simulink model "uz_codegen"  (R2021a)
settings: Solver=FixedStepDiscrete  StartTime=0.0  StopTime=50  RelTol=1e-3  EnableMultiTasking=on
PreLoadFcn:
  | uz_setCodegenPaths
model workspace (MATLAB code in the model file):
  | cmdLim = Simulink.Parameter;
  | cmdLim.Value = 15;
  | cmdLim.Description = 'Limit for controlling the maximum surface command angle.';
  | cmdLim.Min = 0;
  | cmdLim.Max = 90;
  | cmdLim.DocUnits = 'deg';
  | 
  | dispGain = Simulink.Parameter;
  | dispGain.Value = 0.75;
  | dispGain.Description = 'Gain applied to the displacement error.';
  | dispGain.Min = 0;
  | dispGain.Max = [];
  | dispGain.DocUnits = 'deg/sec/deg';
  | 
  | dispLim = Simulink.Parameter;
  | dispLim.Value = 30;
  | dispLim.Description = 'Limit for controlling the maximum commanded angle.';
  | dispLim.Min = 0;
  | dispLim.Max = 180;
  | dispLim.DocUnits = 'deg';
  | 
  | intGain = Simulink.Parameter;
  | intGain.Value = 0.5;
  | intGain.Description = 'Gain applied to the integral error.';
  | intGain.Min = 0;
  | intGain.Max = [];
  | intGain.DocUnits = 'deg/sec/deg/sec';
  | 
  | intLim = Simulink.Parameter;
  | intLim.Value = 5;
  | intLim.Description = 'Limit for controlling the maximum commanded angle.';
  | intLim.Min = 0;
  | intLim.Max = 90;
  | intLim.DocUnits = 'deg';
  | 
  | rateGain = Simulink.Parameter;
  | rateGain.Value = 2;
  | rateGain.Description = 'Gain applied to the rate error.';
  | rateGain.Min = 0;
  | rateGain.Max = [];
  | rateGain.DocUnits = 'deg/deg/sec';
  | 
  | rateLim = Simulink.Parameter;
  | rateLim.Value = 6;
  | rateLim.Description = 'Limit for controlling the maximum commanded angle.';
  | rateLim.Min = 0;
  | rateLim.Max = 180;
  | rateLim.DocUnits = 'deg/sec';
  | 
  | hdgGain = Simulink.Parameter;
  | hdgGain.Value = 0.015;
values from neighbouring files (symbols this model uses):
  I_max = 100    [PMSM_01_Parameter.m]
  Iq_Intersection_Wb = sqrt(I_max^2 - Id_Intersection_Wb^2)    [Plot_MMPA.m]
  Ki_IdController = R/Ld    (= 3749.81250937)    [PMSM_01_Parameter.m]
  Ki_IqController = R/Lq    (= 2500)    [PMSM_01_Parameter.m]
  Ki_SpeedController = Kp_IqController/(Lq*damping_factor^2)    (= 174.532925199)    [PMSM_01_Parameter.m]
  Ki_TorqueController = 1/(4*T_summe_Torque)    (= 714.285714286)    [PMSM_01_Parameter.m]
  Kp_IdController = Ld*2*pi*BW    (= 0.0670239943087)    [PMSM_01_Parameter.m]
  Kp_IqController = Lq*2*pi*BW    (= 0.100530964915)    [PMSM_01_Parameter.m]
  Kp_SpeedController = Kp_IqController/(Lq*damping_factor*K)    (= 2.90111828368)    [PMSM_01_Parameter.m]
  Kp_TorqueController = T1_Torque/(2*T_summe_Torque)    (= 0.373999125427)    [PMSM_01_Parameter.m]
  Ld = 0.6667*Lq    (= 1.06672e-05)    [PMSM_01_Parameter.m]
  List_Iq_Intersection_Speed = zeros(length(List_wEl_Intersection_Speed),1)    [Plot_MMPA.m]
  List_Iq_Torque = zeros(length(List_M_const),1)    [Plot_MMPA.m]
  List_Iq_Torque_Imax = List_Iq_Torque_Imax(List_Iq_Torque_Imax ~= -1)    [Plot_MMPA.m]
  List_M_const = 0:0.5:10    [Plot_MMPA.m]
  List_M_Imax = List_M_const(List_Iq_Torque_Imax ~= -1)    [Plot_MMPA.m]
  List_wEl_Intersection_Speed = linspace(n_cut,n_max,15)    [Plot_MMPA.m]
  Lq = 16e-6    (= 1.6e-05)    [PMSM_01_Parameter.m]
  n_cut = w_b*30/(pi*zp)    [Plot_MMPA.m]
  psi_pm = 0.0030    (= 0.003)    [PMSM_01_Parameter.m]
  R = 0.040    (= 0.04)    [PMSM_01_Parameter.m]
  T_controller = 1/f_CurrentController    (= 0.0001)    [PMSM_01_Parameter.m]
  T_speedController = T_controller    (= 0.0001)    [PMSM_01_Parameter.m]
  U_DC = 46    [PMSM_01_Parameter.m]
  U_maxDQ = U_DC/sqrt(3)    [PMSM_01_Parameter.m]
  zp = 21    [PMSM_01_Parameter.m]
undefined symbols (not defined in the file or in its folder): denum_Gd_speed, denum_Gd_trq, num_Gd_speed, num_Gd_trq
libraries: pid_lib x8, simulink x7, spsabctodq0Lib x2, spsdq0toAlphaBetaZeroLib x2
(part 1 of 2)
settings Model: RequirementInfo={} %GIDa_fe9045fd_0412_4b6e_8206_617cc20e6fde  FPTRunName=Active  Creator=ts  LastModifiedBy=wilflingti66489
settings SolverCC: AlgebraicLoopSolver=TrustRegion  PositivePriorityOrder=on  AutoInsertRateTranBlk=on
settings DataIOCC: SaveOutput=off  SignalLogging=off  DSMLogging=off  SaveTime=off
settings OptimizationCC: DefaultParameterBehavior=Inlined  UseDivisionForNetSlopeComputation=on  GainParamInheritBuiltInType=on  UseFloatMulNetSlope=on  UseSpecifiedMinMax=on  InlineInvariantSignals=on  PassReuseOutputArgsAs=Individual arguments  NoFixptDivByZeroProtection=on  EfficientFloat2IntCast=on  LifeSpan=1  MaxStackSize=64  OptimizeBlockOrder=speed  DifferentSizesBufferReuse=on  EfficientTunableParamExpr=on
settings DebuggingCC: AllowSymbolicDim=off  SFUnexpectedBacktrackingDiag=warning  SFNoUnconditionalDefaultTransitionDiag=warning  SFExecutionAtInitializationDiag=none  SFMachineParentedDataDiag=warning  ArithmeticOperatorsInVariantConditions=warning
settings HardwareCC: ProdBitPerPointer=32  ProdBitPerSizeT=32  ProdBitPerPtrDiffT=32  ProdLargestAtomicInteger=Long  ProdLargestAtomicFloat=Double  ProdWordSize=32  ProdLongLongMode=on  ProdHWDeviceType=ARM Compatible->ARM Cortex-R  HardwareBoardFeatureSet=SoCBlockset
settings SFSimCC: MATLABDynamicMemAlloc=off
settings RTWCC: SystemTargetFile=ert.tlc  GenCodeOnly=on  TemplateMakefile=ert_default_tmf  GenerateReport=on  BuildConfiguration=Faster Runs  IncludeHyperlinkInReport=on  GenerateCodeMetricsReport=on  CheckMdlBeforeBuild=Warning
settings CodeAppCC: ForceParamTrailComments=on  IgnoreCustomStorageClasses=off  OperatorAnnotations=on  SimulinkDataObjDesc=on  SFDataObjDesc=on  MATLABFcnDesc=on  CustomSymbolStrGlobalVar=rt$N$M  CustomSymbolStrType=$N$M  CustomSymbolStrFcn=$N$M$F  CustomSymbolStrMacro=$N$M  InsertBlockDesc=on  StateflowObjectComments=on  MATLABSourceComments=on  EnableCustomComments=on  ReqsInCode=on
settings ERTTargetCC: TargetLangStandard=C99 (ISO)  CodeReplacementLibrary=GNU C99 extensions  MultiwordLength=2048  IncludeMdlTerminateFcn=off  CombineSignalStateStructs=on  SuppressErrorStatus=on  IncludeFileDelimiter=UseQuote  CodeInterfacePackaging=Reusable function  RemoveResetFunc=off  InlinedParameterPlacement=NonHierarchical  MultiInstanceErrorCode=Warning  RootIOFormat=Part of model data structure  ERTCustomFileTemplate=example_file_process.tlc  GlobalDataDefinition=InSourceFile  GlobalDataReference=InSourceFile  ERTFilePackagingFormat=CompactWithDataFile
settings ConfigComp: CovScope=ReferencedModels  CovSaveName=covdata_rollAP  CovMetricSettings=dcmtrwe  CovHTMLOptions=-sRT=1 -aTS=1 -bRG=1 -bTC=1 -hTR=1 -nFC=0 -scm=1 -bcm=1 -xEv=0  CovSaveCumulativeToWorkspaceVar=on  CovSaveSingleToWorkspaceVar=on  CovCumulativeVarName=covCumulativeData_rollAP  CovReportOnPause=off  CovExternalEMLEnable=off  CovSFcnEnable=off

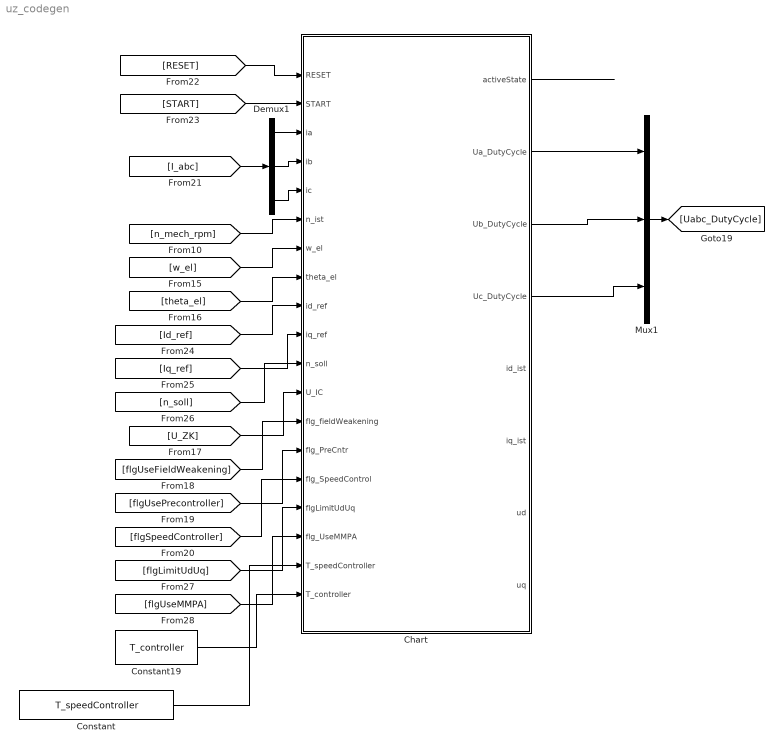
== system uz_codegen ==
  Chart : Stateflow chart  TreatAsAtomicUnit=on
      settings: PortSchema="{\"entries\":[{\"content\":{\"sides\":[{\"content\":{\"connectorIds\":[\"In14\",\"In15\",\"In7\",\"In5\",\"In4\",\"In10\",\"In6\",\"In8\",\"In11\",\"In9\",\"In12\",\"In13\",\"In2\",\"In1\",\"In3\",\"In16\",\"In17\",\"In18\",\"In19\"]},\"type\":\"ConnectorPlacement.EquallySpacedRectSide\",\"uuid\":\"76a4c5fd-8833-454d-a27c-9cb5ddbec7a7\"},{\"content\":{\"connectorIds\":[\"Out2\",\"Out1\",\"Out4\",\"Out3\",\"Out6\",\"Out5\",\"Out8\",\"Out7\"],\"side\":\"RIGHT\"},\"type\":\"ConnectorPlacement.EquallySpacedRectSide\",\"uuid\":\"21c8cff2-6555-410e-8e51-882650c7a948\"},{\"content\":{\"connectorIds\":[],\"side\":\"TOP\"},\"type\":\"ConnectorPlacement.EquallySpacedRectSide\",\"uuid\":\"0c75ee88-c520-42c4-9c42-3a1aac3b64b6\"}]},\"type\":\"ConnectorPlacement.EquallySpacedConnector\",\"uuid\":\"5756a7ca-2edf-4f43-a7f7-e1c56b726d1a\"}],\"packageUris\":[\"http://schema.mathworks.com/mf0/Connector/R2020b\"],\"version\":\"1.0\"}"
  Constant : Constant  Value=T_speedController
  Constant19 : Constant  Value=T_controller
  Demux1 : Demux  Outputs=3
  Mux1 : Mux  Inputs=3
  wires:
  Demux1/3 -> Chart/4(ic)
  [flgUsePrecontroller] -> Chart/1(flg_PreCntr)
  [flgUseMMPA] -> Chart/17(flg_UseMMPA)
  Constant/1 -> Chart/18(T_speedController)
  [flgUseFieldWeakening] -> Chart/2(flg_fieldWeakening)
  Chart/3(Uc_DutyCycle) -> Mux1/3
  [w_el] -> Chart/6(w_el)
  [flgLimitUdUq] -> Chart/16(flgLimitUdUq)
  [n_mech_rpm] -> Chart/10(n_ist)
  [U_ZK] -> Chart/13(U_IC)
  Chart/4(Ub_DutyCycle) -> Mux1/2
  Demux1/1 -> Chart/7(ia)
  Chart/2(activeState) -> ?
  [Iq_ref] -> Chart/9(iq_ref)
  [n_soll] -> Chart/12(n_soll)
  Mux1/1 -> [Uabc_DutyCycle]
  Constant19/1 -> Chart/19(T_controller)
  [theta_el] -> Chart/8(theta_el)
  [flgSpeedController] -> Chart/3(flg_SpeedControl)
  [I_abc] -> Demux1/1
  Chart/1(Ua_DutyCycle) -> Mux1/1
  [START] -> Chart/15(START)
  Demux1/2 -> Chart/5(ib)
  [RESET] -> Chart/14(RESET)
  [Id_ref] -> Chart/11(id_ref)

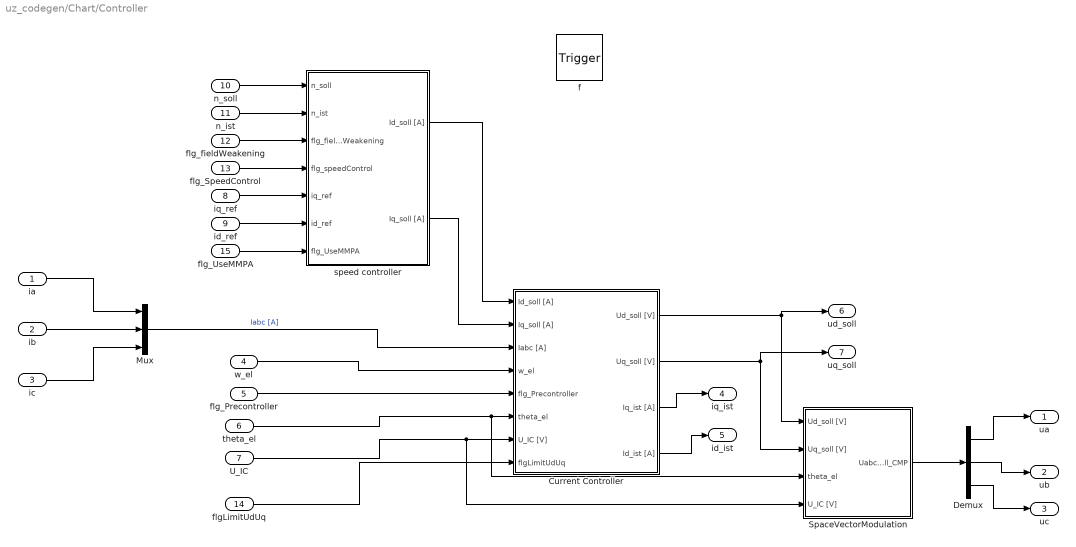
== system uz_codegen/Chart/Controller ==
  ia : Inport  OutDataTypeStr=double  PortDimensions=1
  ib : Inport  Port=2  OutDataTypeStr=double  PortDimensions=1
  ic : Inport  Port=3  OutDataTypeStr=double  PortDimensions=1
  w_el : Inport  Port=4  OutDataTypeStr=double  PortDimensions=1
  flg_Precontroller : Inport  Port=5  OutDataTypeStr=double  PortDimensions=1
  theta_el : Inport  Port=6  OutDataTypeStr=double  PortDimensions=1
  U_IC : Inport  Port=7  OutDataTypeStr=double  PortDimensions=1
  iq_ref : Inport  Port=8  OutDataTypeStr=double  PortDimensions=1
  id_ref : Inport  Port=9  OutDataTypeStr=double  PortDimensions=1
  n_soll : Inport  Port=10  OutDataTypeStr=double  PortDimensions=1
  n_ist : Inport  Port=11  OutDataTypeStr=double  PortDimensions=1
  flg_fieldWeakening : Inport  Port=12  OutDataTypeStr=double  PortDimensions=1
  flg_SpeedControl : Inport  Port=13  OutDataTypeStr=double  PortDimensions=1
  flgLimitUdUq : Inport  Port=14  OutDataTypeStr=double  PortDimensions=1
  flg_UseMMPA : Inport  Port=15  OutDataTypeStr=double  PortDimensions=1
  f : TriggerPort  TriggerType=function-call  VariantControl=(inherit)
      settings: CopyFcn=Stateflow.SLINSF.SimulinkMan.removeBlockPreDeleteFcn  PreDeleteFcn=Stateflow.SLINSF.SimulinkMan.unsafePredeleteFcn
  Current Controller : Subsystem
  Demux : Demux  Outputs=3
  Mux : Mux  Inputs=3
  SpaceVectorModulation : Subsystem
  speed controller : Subsystem
  ua : Outport
  ub : Outport  Port=2
  uc : Outport  Port=3
  iq_ist : Outport  Port=4
  id_ist : Outport  Port=5
  ud_soll : Outport  Port=6
  uq_soll : Outport  Port=7
  wires:
  Current Controller/2(Uq_soll [V]) -> uq_soll/1, SpaceVectorModulation/2(Uq_soll [V])
  speed controller/1(Id_soll [A]) -> Current Controller/1(Id_soll [A])
  Current Controller/1(Ud_soll [V]) -> ud_soll/1, SpaceVectorModulation/1(Ud_soll [V])
  speed controller/2(Iq_soll [A]) -> Current Controller/2(Iq_soll [A])
  SpaceVectorModulation/1(Uabc_soll_CMP) -> Demux/1
  Demux/1 -> ua/1
  Demux/2 -> ub/1
  Demux/3 -> uc/1
  Current Controller/3(Iq_ist [A]) -> iq_ist/1
  Current Controller/4(Id_ist [A]) -> id_ist/1
  ic/1 -> Mux/3
  ib/1 -> Mux/2
  ia/1 -> Mux/1
  Mux/1 -> Current Controller/3(Iabc [A])  "Iabc [A]"
  w_el/1 -> Current Controller/4(w_el)
  flg_Precontroller/1 -> Current Controller/5(flg_Precontroller)
  theta_el/1 -> SpaceVectorModulation/3(theta_el), Current Controller/6(theta_el)
  U_IC/1 -> SpaceVectorModulation/4(U_IC [V]), Current Controller/7(U_IC [V])
  iq_ref/1 -> speed controller/5(iq_ref)
  id_ref/1 -> speed controller/6(id_ref)
  n_soll/1 -> speed controller/1(n_soll)
  n_ist/1 -> speed controller/2(n_ist)
  flg_fieldWeakening/1 -> speed controller/3(flg_fieldWeakening)
  flg_SpeedControl/1 -> speed controller/4(flg_speedControl)
  flgLimitUdUq/1 -> Current Controller/8(flgLimitUdUq)
  flg_UseMMPA/1 -> speed controller/7(flg_UseMMPA)

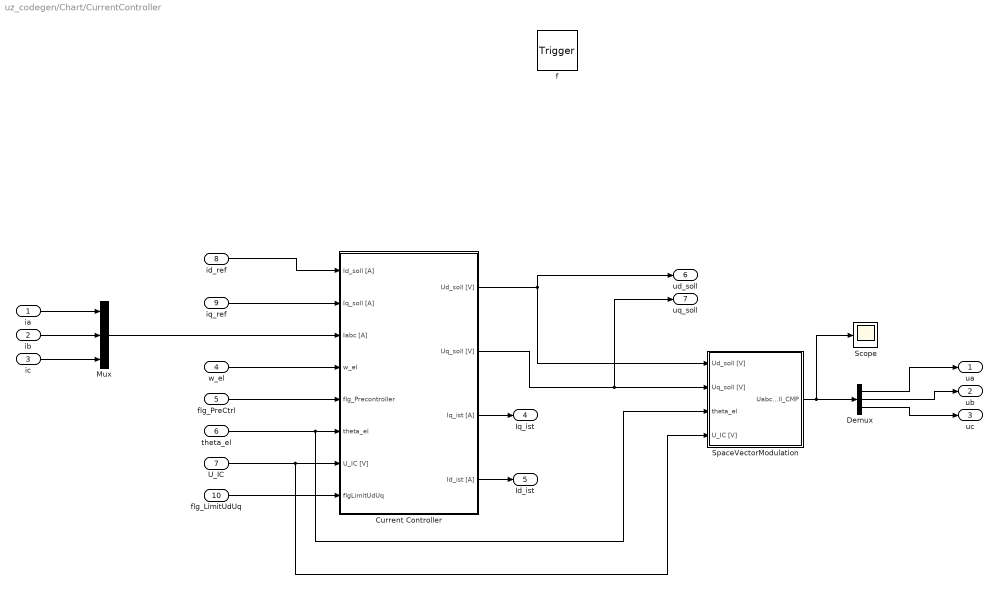
== system uz_codegen/Chart/CurrentController ==
  ia : Inport  OutDataTypeStr=double  PortDimensions=1
  ib : Inport  Port=2  OutDataTypeStr=double  PortDimensions=1
  ic : Inport  Port=3  OutDataTypeStr=double  PortDimensions=1
  w_el : Inport  Port=4  OutDataTypeStr=double  PortDimensions=1
  flg_PreCtrl : Inport  Port=5  OutDataTypeStr=double  PortDimensions=1
  theta_el : Inport  Port=6  OutDataTypeStr=double  PortDimensions=1
  U_IC : Inport  Port=7  OutDataTypeStr=double  PortDimensions=1
  id_ref : Inport  Port=8  OutDataTypeStr=double  PortDimensions=1
  iq_ref : Inport  Port=9  OutDataTypeStr=double  PortDimensions=1
  flg_LimitUdUq : Inport  Port=10  OutDataTypeStr=double  PortDimensions=1
  f : TriggerPort  TriggerType=function-call  VariantControl=(inherit)
      settings: CopyFcn=Stateflow.SLINSF.SimulinkMan.removeBlockPreDeleteFcn  PreDeleteFcn=Stateflow.SLINSF.SimulinkMan.unsafePredeleteFcn
  Current Controller : Subsystem
  Demux : Demux  Outputs=3
  Mux : Mux  Inputs=3
  Scope : Scope
  SpaceVectorModulation : Subsystem
  ua : Outport
  ub : Outport  Port=2
  uc : Outport  Port=3
  Iq_ist : Outport  Port=4
  Id_ist : Outport  Port=5
  ud_soll : Outport  Port=6
  uq_soll : Outport  Port=7
  wires:
  Current Controller/2(Uq_soll [V]) -> uq_soll/1, SpaceVectorModulation/2(Uq_soll [V])
  id_ref/1 -> Current Controller/1(Id_soll [A])
  iq_ref/1 -> Current Controller/2(Iq_soll [A])
  w_el/1 -> Current Controller/4(w_el)
  flg_LimitUdUq/1 -> Current Controller/8(flgLimitUdUq)
  U_IC/1 -> SpaceVectorModulation/4(U_IC [V]), Current Controller/7(U_IC [V])
  theta_el/1 -> SpaceVectorModulation/3(theta_el), Current Controller/6(theta_el)
  flg_PreCtrl/1 -> Current Controller/5(flg_Precontroller)
  ib/1 -> Mux/2
  ia/1 -> Mux/1
  ic/1 -> Mux/3
  Mux/1 -> Current Controller/3(Iabc [A])
  Current Controller/3(Iq_ist [A]) -> Iq_ist/1
  Current Controller/4(Id_ist [A]) -> Id_ist/1
  SpaceVectorModulation/1(Uabc_soll_CMP) -> Scope/1, Demux/1
  Demux/1 -> ua/1
  Demux/2 -> ub/1
  Demux/3 -> uc/1
  Current Controller/1(Ud_soll [V]) -> SpaceVectorModulation/1(Ud_soll [V]), ud_soll/1

== system uz_codegen/Chart/SpeedController ==
  id_ref : Inport  OutDataTypeStr=double  PortDimensions=1
  iq_ref : Inport  Port=2  OutDataTypeStr=double  PortDimensions=1
  n_soll : Inport  Port=3  OutDataTypeStr=double  PortDimensions=1
  n_ist : Inport  Port=4  OutDataTypeStr=double  PortDimensions=1
  flg_fieldWeakening : Inport  Port=5  OutDataTypeStr=double  PortDimensions=1
  flg_UseMMPA : Inport  Port=6  OutDataTypeStr=double  PortDimensions=1
  flg_SpeedControl : Inport  Port=7  OutDataTypeStr=double  PortDimensions=1
  f : TriggerPort  TriggerType=function-call  VariantControl=(inherit)
      settings: CopyFcn=Stateflow.SLINSF.SimulinkMan.removeBlockPreDeleteFcn  PreDeleteFcn=Stateflow.SLINSF.SimulinkMan.unsafePredeleteFcn
  Scope : Scope  NumInputPorts=2
  speed controller : Subsystem
  id_soll : Outport
  iq_soll : Outport  Port=2
  wires:
  flg_SpeedControl/1 -> speed controller/7(flg_speedControl)
  flg_UseMMPA/1 -> speed controller/6(flg_UseMMPA)
  flg_fieldWeakening/1 -> speed controller/5(flg_fieldWeakening)
  n_ist/1 -> speed controller/4(n_ist)
  n_soll/1 -> speed controller/3(n_soll)
  iq_ref/1 -> speed controller/2(iq_ref)
  id_ref/1 -> speed controller/1(id_ref)
  speed controller/1(Id_soll [A]) -> Scope/1, id_soll/1
  speed controller/2(Iq_soll [A]) -> Scope/2, iq_soll/1

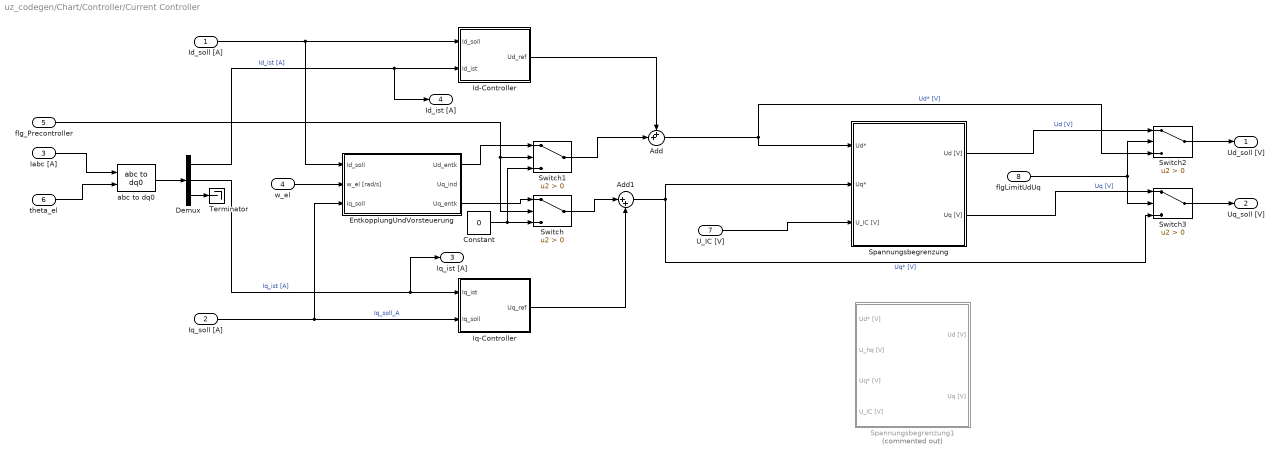
== system uz_codegen/Chart/Controller/Current Controller ==
  Id_soll [A] : Inport
  Iq_soll [A] : Inport  Port=2
  Iabc [A] : Inport  Port=3
  w_el : Inport  Port=4
  flg_Precontroller : Inport  Port=5
  theta_el : Inport  Port=6
  U_IC [V] : Inport  Port=7
  flgLimitUdUq : Inport  Port=8
  Add : Sum  Inputs=++|
  Add1 : Sum  Inputs=|++
  Constant : Constant  Value=0
  Demux : Demux  Outputs=3
  EntkopplungUndVorsteuerung : Subsystem
  Id-Controller : Subsystem
  Iq-Controller : Subsystem
  Spannungsbegrenzung : Subsystem
  Spannungsbegrenzung1 : Subsystem  Commented=on
  Switch{,1..3} (4 alike) : Switch  Criteria=u2 > Threshold
  Terminator : Terminator
  abc to dq0 : spsabctodq0Lib/abc to dq0  Alignment=Aligned with phase A axis
  Ud_soll [V] : Outport
  Uq_soll [V] : Outport  Port=2
  Iq_ist [A] : Outport  Port=3
  Id_ist [A] : Outport  Port=4
  wires:
  Add1/1 -> Switch3/3, Spannungsbegrenzung/2(Uq*)  "Uq* [V]"
  Add/1 -> Switch2/3, Spannungsbegrenzung/1(Ud*)  "Ud* [V]"
  Id_soll [A]/1 -> EntkopplungUndVorsteuerung/1(Id_soll), Id-Controller/1(Id_soll)
  Iabc [A]/1 -> abc to dq0/1
  theta_el/1 -> abc to dq0/2
  abc to dq0/1 -> Demux/1
  Demux/1 -> Id_ist [A]/1, Id-Controller/2(Id_ist)  "Id_ist [A]"
  Demux/2 -> Iq_ist [A]/1, Iq-Controller/1(Iq_ist)  "Iq_ist [A]"
  Demux/3 -> Terminator/1
  w_el/1 -> EntkopplungUndVorsteuerung/2(w_el [rad/s])
  EntkopplungUndVorsteuerung/3(Uq_entk) -> Switch/1
  EntkopplungUndVorsteuerung/1(Ud_entk) -> Switch1/1
  Constant/1 -> Switch1/3, Switch/3
  flg_Precontroller/1 -> Switch/2, Switch1/2
  Iq-Controller/1(Uq_ref) -> Add1/2
  Iq_soll [A]/1 -> EntkopplungUndVorsteuerung/3(Iq_soll), Iq-Controller/2(Iq_soll)  "Iq_soll_A"
  U_IC [V]/1 -> Spannungsbegrenzung/3(U_IC [V])
  Spannungsbegrenzung/1(Ud [V]) -> Switch2/1  "Ud [V]"
  Spannungsbegrenzung/2(Uq [V]) -> Switch3/1  "Uq [V]"
  Switch1/1 -> Add/2
  Switch/1 -> Add1/1
  Id-Controller/1(Ud_ref) -> Add/1
  Switch2/1 -> Ud_soll [V]/1
  Switch3/1 -> Uq_soll [V]/1
  flgLimitUdUq/1 -> Switch3/2, Switch2/2

== system uz_codegen/Chart/Controller/SpaceVectorModulation ==
  Ud_soll [V] : Inport
  Uq_soll [V] : Inport  Port=2
  theta_el : Inport  Port=3
  U_IC [V] : Inport  Port=4
  Constant : Constant  Value=0
  Demux : Demux  Outputs=3
  Mux : Mux  Inputs=3
  Mux2 : Mux  Inputs=3
  SpaceVectorModulation : MATLAB Function  TreatAsAtomicUnit=on
  Terminator : Terminator
  dq0 to Alpha-Beta-Zero : spsdq0toAlphaBetaZeroLib/dq0 to Alpha-Beta-Zero  Alignment=Aligned with phase A axis
      settings: SourceProductBaseCode=PS
  Uabc_soll_CMP : Outport
  wires:
  Ud_soll [V]/1 -> Mux/1
  Uq_soll [V]/1 -> Mux/2
  Constant/1 -> Mux/3
  Mux/1 -> dq0 to Alpha-Beta-Zero/1  "Udq0 [V]"
  theta_el/1 -> dq0 to Alpha-Beta-Zero/2
  Demux/1 -> SpaceVectorModulation/1(u_alpha)
  Demux/2 -> SpaceVectorModulation/2(u_beta)
  Demux/3 -> Terminator/1
  SpaceVectorModulation/1(u_a) -> Mux2/1
  SpaceVectorModulation/2(u_b) -> Mux2/2
  SpaceVectorModulation/3(u_c) -> Mux2/3
  dq0 to Alpha-Beta-Zero/1 -> Demux/1  "UalphaBeta [V]"
  Mux2/1 -> Uabc_soll_CMP/1  "Uabc_soll_CMP"
  U_IC [V]/1 -> SpaceVectorModulation/3(U_ZK)

== system uz_codegen/Chart/Controller/speed controller ==
  n_soll : Inport
  n_ist : Inport  Port=2
  flg_fieldWeakening : Inport  Port=3
  flg_speedControl : Inport  Port=4
  iq_ref : Inport  Port=5
  id_ref : Inport  Port=6
  flg_UseMMPA : Inport  Port=7
  MMPA_Controller : Subsystem
  Subsystem : Subsystem
  Switch : Switch  Criteria=u2 > Threshold
  Switch1 : Switch  Criteria=u2 > Threshold
  Id_soll [A] : Outport
  Iq_soll [A] : Outport  Port=2
  wires:
  flg_fieldWeakening/1 -> Subsystem/1(flg_fieldWeakening)
  id_ref/1 -> MMPA_Controller/4(id_ref), Subsystem/2(id_ref)
  flg_speedControl/1 -> MMPA_Controller/1(flg_speedControl), Subsystem/4(flg_speedControl)
  n_ist/1 -> MMPA_Controller/3(n_ist), Subsystem/5(n_ist)
  iq_ref/1 -> MMPA_Controller/5(iq_ref), Subsystem/6(iq_ref)
  Subsystem/1(id_soll) -> Switch/3
  Subsystem/2(iq_soll) -> Switch1/3
  MMPA_Controller/1(id_soll) -> Switch/1
  Switch/1 -> Id_soll [A]/1
  Switch1/1 -> Iq_soll [A]/1
  MMPA_Controller/2(Iq_soll) -> Switch1/1
  flg_UseMMPA/1 -> Switch/2, Switch1/2
  n_soll/1 -> MMPA_Controller/2(n_soll), Subsystem/3(n_soll)

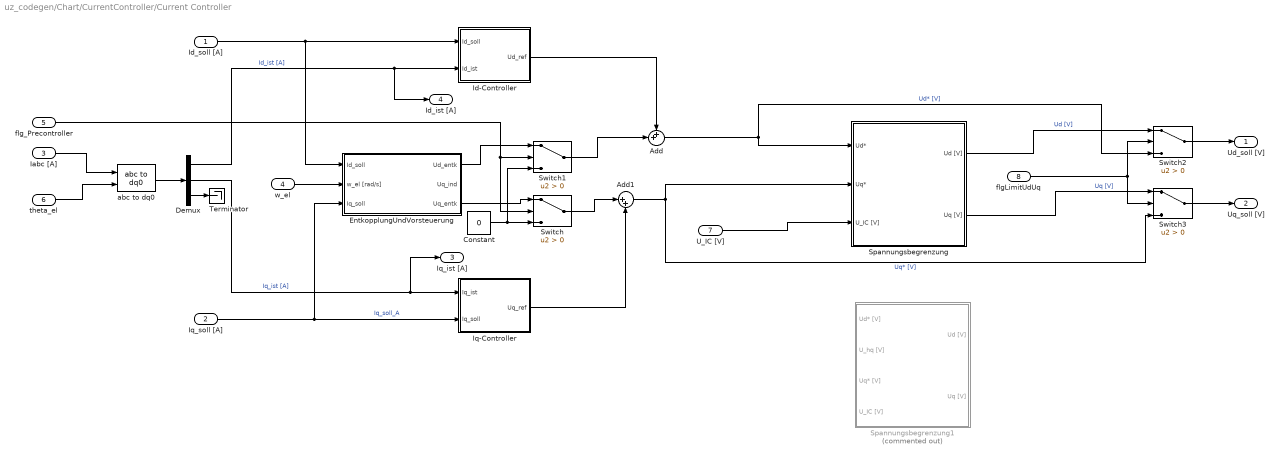
== system uz_codegen/Chart/CurrentController/Current Controller ==
  Id_soll [A] : Inport
  Iq_soll [A] : Inport  Port=2
  Iabc [A] : Inport  Port=3
  w_el : Inport  Port=4
  flg_Precontroller : Inport  Port=5
  theta_el : Inport  Port=6
  U_IC [V] : Inport  Port=7
  flgLimitUdUq : Inport  Port=8
  Add : Sum  Inputs=++|
  Add1 : Sum  Inputs=|++
  Constant : Constant  Value=0
  Demux : Demux  Outputs=3
  EntkopplungUndVorsteuerung : Subsystem
  Id-Controller : Subsystem
  Iq-Controller : Subsystem
  Spannungsbegrenzung : Subsystem
  Spannungsbegrenzung1 : Subsystem  Commented=on
  Switch{,1..3} (4 alike) : Switch  Criteria=u2 > Threshold
  Terminator : Terminator
  abc to dq0 : spsabctodq0Lib/abc to dq0  Alignment=Aligned with phase A axis
  Ud_soll [V] : Outport
  Uq_soll [V] : Outport  Port=2
  Iq_ist [A] : Outport  Port=3
  Id_ist [A] : Outport  Port=4
  wires:
  Add1/1 -> Switch3/3, Spannungsbegrenzung/2(Uq*)  "Uq* [V]"
  Add/1 -> Switch2/3, Spannungsbegrenzung/1(Ud*)  "Ud* [V]"
  Id_soll [A]/1 -> EntkopplungUndVorsteuerung/1(Id_soll), Id-Controller/1(Id_soll)
  Iabc [A]/1 -> abc to dq0/1
  theta_el/1 -> abc to dq0/2
  abc to dq0/1 -> Demux/1
  Demux/1 -> Id_ist [A]/1, Id-Controller/2(Id_ist)  "Id_ist [A]"
  Demux/2 -> Iq_ist [A]/1, Iq-Controller/1(Iq_ist)  "Iq_ist [A]"
  Demux/3 -> Terminator/1
  w_el/1 -> EntkopplungUndVorsteuerung/2(w_el [rad/s])
  EntkopplungUndVorsteuerung/3(Uq_entk) -> Switch/1
  EntkopplungUndVorsteuerung/1(Ud_entk) -> Switch1/1
  Constant/1 -> Switch1/3, Switch/3
  flg_Precontroller/1 -> Switch/2, Switch1/2
  Iq-Controller/1(Uq_ref) -> Add1/2
  Iq_soll [A]/1 -> EntkopplungUndVorsteuerung/3(Iq_soll), Iq-Controller/2(Iq_soll)  "Iq_soll_A"
  U_IC [V]/1 -> Spannungsbegrenzung/3(U_IC [V])
  Spannungsbegrenzung/1(Ud [V]) -> Switch2/1  "Ud [V]"
  Spannungsbegrenzung/2(Uq [V]) -> Switch3/1  "Uq [V]"
  Switch1/1 -> Add/2
  Switch/1 -> Add1/1
  Id-Controller/1(Ud_ref) -> Add/1
  Switch2/1 -> Ud_soll [V]/1
  Switch3/1 -> Uq_soll [V]/1
  flgLimitUdUq/1 -> Switch3/2, Switch2/2

== system uz_codegen/Chart/CurrentController/SpaceVectorModulation ==
  Ud_soll [V] : Inport
  Uq_soll [V] : Inport  Port=2
  theta_el : Inport  Port=3
  U_IC [V] : Inport  Port=4
  Constant : Constant  Value=0
  Demux : Demux  Outputs=3
  Mux : Mux  Inputs=3
  Mux2 : Mux  Inputs=3
  SpaceVectorModulation : MATLAB Function  TreatAsAtomicUnit=on
  Terminator : Terminator
  dq0 to Alpha-Beta-Zero : spsdq0toAlphaBetaZeroLib/dq0 to Alpha-Beta-Zero  Alignment=Aligned with phase A axis
      settings: SourceProductBaseCode=PS
  Uabc_soll_CMP : Outport
  wires:
  Ud_soll [V]/1 -> Mux/1
  Uq_soll [V]/1 -> Mux/2
  Constant/1 -> Mux/3
  Mux/1 -> dq0 to Alpha-Beta-Zero/1  "Udq0 [V]"
  theta_el/1 -> dq0 to Alpha-Beta-Zero/2
  Demux/1 -> SpaceVectorModulation/1(u_alpha)
  Demux/2 -> SpaceVectorModulation/2(u_beta)
  Demux/3 -> Terminator/1
  SpaceVectorModulation/1(u_a) -> Mux2/1
  SpaceVectorModulation/2(u_b) -> Mux2/2
  SpaceVectorModulation/3(u_c) -> Mux2/3
  dq0 to Alpha-Beta-Zero/1 -> Demux/1  "UalphaBeta [V]"
  Mux2/1 -> Uabc_soll_CMP/1  "Uabc_soll_CMP"
  U_IC [V]/1 -> SpaceVectorModulation/3(U_ZK)

== system uz_codegen/Chart/SpeedController/speed controller ==
  id_ref : Inport
  iq_ref : Inport  Port=2
  n_soll : Inport  Port=3
  n_ist : Inport  Port=4
  flg_fieldWeakening : Inport  Port=5
  flg_UseMMPA : Inport  Port=6
  flg_speedControl : Inport  Port=7
  MMPA_Controller : Subsystem
  Subsystem : Subsystem
  Switch : Switch  Criteria=u2 > Threshold
  Switch1 : Switch  Criteria=u2 > Threshold
  Id_soll [A] : Outport
  Iq_soll [A] : Outport  Port=2
  wires:
  flg_fieldWeakening/1 -> Subsystem/1(flg_fieldWeakening)
  id_ref/1 -> MMPA_Controller/4(id_ref), Subsystem/2(id_ref)
  flg_speedControl/1 -> MMPA_Controller/1(flg_speedControl), Subsystem/4(flg_speedControl)
  n_ist/1 -> MMPA_Controller/3(n_ist), Subsystem/5(n_ist)
  iq_ref/1 -> MMPA_Controller/5(iq_ref), Subsystem/6(iq_ref)
  Subsystem/1(id_soll) -> Switch/3
  Subsystem/2(iq_soll) -> Switch1/3
  MMPA_Controller/1(id_soll) -> Switch/1
  Switch/1 -> Id_soll [A]/1
  Switch1/1 -> Iq_soll [A]/1
  MMPA_Controller/2(Iq_soll) -> Switch1/1
  flg_UseMMPA/1 -> Switch/2, Switch1/2
  n_soll/1 -> MMPA_Controller/2(n_soll), Subsystem/3(n_soll)

== system uz_codegen/Chart/Controller/Current Controller/EntkopplungUndVorsteuerung ==
  Id_soll : Inport
  w_el [rad/s] : Inport  Port=2
  Iq_soll : Inport  Port=3
  Add : Sum
  Constant : Constant  Value=psi_pm
  Gain1 : Gain  Gain=-Lq
  Gain2 : Gain  Gain=Ld
  Product : Product
  Product1 : Product
  Product2 : Product
  Ud_entk : Outport
  Uq_ind : Outport  Port=2
  Uq_entk : Outport  Port=3
  wires:
  w_el [rad/s]/1 -> Product2/2, Product1/2, Product/1  "w_el [rad/s]"
  Iq_soll/1 -> Gain1/1
  Gain1/1 -> Product/2
  Product/1 -> Ud_entk/1  "-w_el * Iq * Lq"
  Id_soll/1 -> Gain2/1
  Gain2/1 -> Add/2
  Constant/1 -> Product2/1, Add/1
  Add/1 -> Product1/1
  Product1/1 -> Uq_entk/1  "w_el * (psi_pm + Ld * Id)"
  Product2/1 -> Uq_ind/1

== system uz_codegen/Chart/Controller/Current Controller/Id-Controller ==
  Id_soll : Inport
  Id_ist : Inport  Port=2
  PID Controller : pid_lib/PID Controller  Controller=PI  Form=Ideal  TimeDomain=Discrete-time  UseExternalTs=off  SampleTime=-1  IntegratorMethod=Forward Euler  FilterMethod=Forward Euler  ControllerParametersSource=internal  P=Kp_IdController  I=Ki_IdController  D=0  UseFilter=on  N=100  TunerSelectOption=Transfer Function Based (PID Tuner App)  InitialConditionSource=internal  InitialConditionForIntegrator=0  InitialConditionForFilter=0  DifferentiatorICPrevScaledInput=0  ExternalReset=none  TrackingMode=off  Kt=1  LimitOutput=on  SatLimitsSource=internal  UpperSaturationLimit=U_maxDQ  LowerSaturationLimit=-U_maxDQ  LinearizeAsGain=on  AntiWindupMode=clamping  Kb=1  POutMin=[]  POutMax=[]  IOutMin=[]  IOutMax=[]  DOutMin=[]  DOutMax=[]  NOutMin=[]  NOutMax=[]  SumOutMin=[]  SumOutMax=[]  SaturationOutMin=[]  SaturationOutMax=[]  PParamMin=[]  PParamMax=[]  IParamMin=[]  IParamMax=[]  DParamMin=[]  DParamMax=[]  NParamMin=[]  NParamMax=[]  KbParamMin=[]  KbParamMax=[]  KtParamMin=[]  KtParamMax=[]  KbOutMin=[]  KbOutMax=[]  KtOutMin=[]  KtOutMax=[]  IntegratorOutMin=[]  IntegratorOutMax=[]  FilterOutMin=[]  FilterOutMax=[]  SumI1OutMin=[]  SumI1OutMax=[]  SumI2OutMin=[]  SumI2OutMax=[]  SumI3OutMin=[]  SumI3OutMax=[]  SumI4OutMin=[]  SumI4OutMax=[]  SumDOutMin=[]  SumDOutMax=[]  DifferentiatorOutMin=[]  DifferentiatorOutMax=[]  FilterDiffOutCoefMin=[]  FilterDiffOutCoefMax=[]  ReciprocalOutMin=[]  ReciprocalOutMax=[]  SumDenOutMin=[]  SumDenOutMax=[]  SumNumOutMin=[]  SumNumOutMax=[]  DivideOutMin=[]  DivideOutMax=[]  UdiffTsProdOutMin=[]  UdiffTsProdOutMax=[]  NTsProdOutMin=[]  NTsProdOutMax=[]  UintegralTsProdOutMin=[]  UintegralTsProdOutMax=[]  UngainTsProdOutMin=[]  UngainTsProdOutMax=[]  IntegratorContinuousStateAttributes=''  IntegratorStateMustResolveToSignalObject=off  IntegratorRTWStateStorageClass=Auto  FilterContinuousStateAttributes=''  FilterStateMustResolveToSignalObject=off  FilterRTWStateStorageClass=Auto  ParallelPVariant=Passthrough  IdealPVariant=InternalParameters  IVariant=InternalParameters  DVariant=Disabled  IntegratorVariant=Discrete  SatVariant=Enabled  AWVariant=DiscClampingIdeal  PCopyVariant=InternalParamsIdeal  TRVariant=Disabled  FdbkBlocksVariant=Forward  IdealPFdbkVariant=Disabled  SatFdbkVariant=Disabled  DerivativeFilterVariant=Disabled  NVariant=Disabled  NCopyVariant=Disabled_SignalSpec  FilterICVariant=Disabled  IntegratorICVariant=InternalICs  ExternalResetVariant=Disabled  TRSumVariant=Passthrough  SumFdbkVariant=Disabled  SumVariant=Sum_PI  TsampFilterVariant=InternalTs  TsampNgainVariant=Passthrough  TsampIntegralVariant=Passthrough  ExternalSaturationOutDataTypeStr=Inherit: Same as second input
  Scope : Scope  NumInputPorts=2
  Subtract : Sum  Inputs=|+-
  Ud_ref : Outport
  wires:
  Subtract/1 -> PID Controller/1  "error"
  Id_soll/1 -> Scope/1, Subtract/1  "id_soll"
  Id_ist/1 -> Scope/2, Subtract/2  "id_ist"
  PID Controller/1 -> Ud_ref/1

== system uz_codegen/Chart/Controller/Current Controller/Iq-Controller ==
  Iq_ist : Inport
  Iq_soll : Inport  Port=2
  PID Controller : pid_lib/PID Controller  Controller=PI  Form=Ideal  TimeDomain=Discrete-time  UseExternalTs=off  SampleTime=-1  IntegratorMethod=Forward Euler  FilterMethod=Forward Euler  ControllerParametersSource=internal  P=Kp_IqController  I=Ki_IqController  D=0  UseFilter=on  N=100  TunerSelectOption=Transfer Function Based (PID Tuner App)  InitialConditionSource=internal  InitialConditionForIntegrator=0  InitialConditionForFilter=0  DifferentiatorICPrevScaledInput=0  ExternalReset=none  TrackingMode=off  Kt=1  LimitOutput=on  SatLimitsSource=internal  UpperSaturationLimit=U_maxDQ  LowerSaturationLimit=-U_maxDQ  LinearizeAsGain=on  AntiWindupMode=clamping  Kb=1  POutMin=[]  POutMax=[]  IOutMin=[]  IOutMax=[]  DOutMin=[]  DOutMax=[]  NOutMin=[]  NOutMax=[]  SumOutMin=[]  SumOutMax=[]  SaturationOutMin=[]  SaturationOutMax=[]  PParamMin=[]  PParamMax=[]  IParamMin=[]  IParamMax=[]  DParamMin=[]  DParamMax=[]  NParamMin=[]  NParamMax=[]  KbParamMin=[]  KbParamMax=[]  KtParamMin=[]  KtParamMax=[]  KbOutMin=[]  KbOutMax=[]  KtOutMin=[]  KtOutMax=[]  IntegratorOutMin=[]  IntegratorOutMax=[]  FilterOutMin=[]  FilterOutMax=[]  SumI1OutMin=[]  SumI1OutMax=[]  SumI2OutMin=[]  SumI2OutMax=[]  SumI3OutMin=[]  SumI3OutMax=[]  SumI4OutMin=[]  SumI4OutMax=[]  SumDOutMin=[]  SumDOutMax=[]  DifferentiatorOutMin=[]  DifferentiatorOutMax=[]  FilterDiffOutCoefMin=[]  FilterDiffOutCoefMax=[]  ReciprocalOutMin=[]  ReciprocalOutMax=[]  SumDenOutMin=[]  SumDenOutMax=[]  SumNumOutMin=[]  SumNumOutMax=[]  DivideOutMin=[]  DivideOutMax=[]  UdiffTsProdOutMin=[]  UdiffTsProdOutMax=[]  NTsProdOutMin=[]  NTsProdOutMax=[]  UintegralTsProdOutMin=[]  UintegralTsProdOutMax=[]  UngainTsProdOutMin=[]  UngainTsProdOutMax=[]  IntegratorContinuousStateAttributes=''  IntegratorStateMustResolveToSignalObject=off  IntegratorRTWStateStorageClass=Auto  FilterContinuousStateAttributes=''  FilterStateMustResolveToSignalObject=off  FilterRTWStateStorageClass=Auto  ParallelPVariant=Passthrough  IdealPVariant=InternalParameters  IVariant=InternalParameters  DVariant=Disabled  IntegratorVariant=Discrete  SatVariant=Enabled  AWVariant=DiscClampingIdeal  PCopyVariant=InternalParamsIdeal  TRVariant=Disabled  FdbkBlocksVariant=Forward  IdealPFdbkVariant=Disabled  SatFdbkVariant=Disabled  DerivativeFilterVariant=Disabled  NVariant=Disabled  NCopyVariant=Disabled_SignalSpec  FilterICVariant=Disabled  IntegratorICVariant=InternalICs  ExternalResetVariant=Disabled  TRSumVariant=Passthrough  SumFdbkVariant=Disabled  SumVariant=Sum_PI  TsampFilterVariant=InternalTs  TsampNgainVariant=Passthrough  TsampIntegralVariant=Passthrough  ExternalSaturationOutDataTypeStr=Inherit: Same as second input
  Scope : Scope  NumInputPorts=2
  Subtract : Sum  Inputs=|+-
  Uq_ref : Outport
  wires:
  Subtract/1 -> PID Controller/1  "error"
  Iq_soll/1 -> Scope/1, Subtract/1  "iq_soll"
  Iq_ist/1 -> Scope/2, Subtract/2  "iq_ist"
  PID Controller/1 -> Uq_ref/1

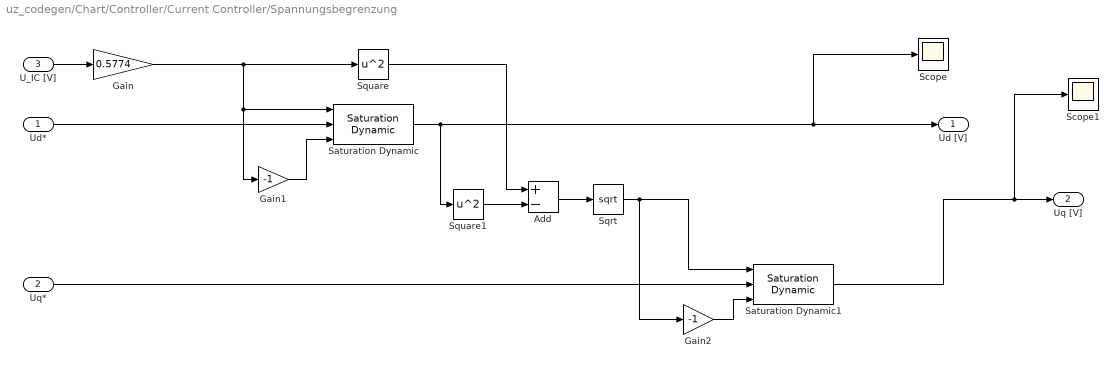
== system uz_codegen/Chart/Controller/Current Controller/Spannungsbegrenzung ==
  Ud* : Inport
  Uq* : Inport  Port=2
  U_IC [V] : Inport  Port=3
  Add : Sum  Inputs=+-
  Gain : Gain  Gain=0.5774
  Gain1 : Gain  Gain=-1
  Gain2 : Gain  Gain=-1
  Saturation Dynamic : simulink/Discontinuities/Saturation Dynamic  OutMin=[]  OutMax=[]  OutDataTypeStr=Inherit: Same as second input  OutDataType=fixdt(1, 16)  OutScaling=2^-10  DoSatur=off
  Saturation Dynamic1 : simulink/Discontinuities/Saturation Dynamic  OutMin=[]  OutMax=[]  OutDataTypeStr=Inherit: Same as second input  OutDataType=fixdt(1, 16)  OutScaling=2^-10  DoSatur=off
  Scope : Scope
  Scope1 : Scope
  Sqrt : Sqrt  SaturateOnIntegerOverflow=on
  Square : Math  Operator=square  SaturateOnIntegerOverflow=on
  Square1 : Math  Operator=square  SaturateOnIntegerOverflow=on
  Ud [V] : Outport
  Uq [V] : Outport  Port=2
  wires:
  Gain2/1 -> Saturation Dynamic1/3
  Add/1 -> Sqrt/1
  Square/1 -> Add/1
  Sqrt/1 -> Gain2/1, Saturation Dynamic1/1
  Saturation Dynamic/1 -> Scope/1, Ud [V]/1, Square1/1
  Saturation Dynamic1/1 -> Scope1/1, Uq [V]/1
  Gain1/1 -> Saturation Dynamic/3
  Uq*/1 -> Saturation Dynamic1/2
  U_IC [V]/1 -> Gain/1
  Gain/1 -> Square/1, Saturation Dynamic/1, Gain1/1
  Square1/1 -> Add/2
  Ud*/1 -> Saturation Dynamic/2

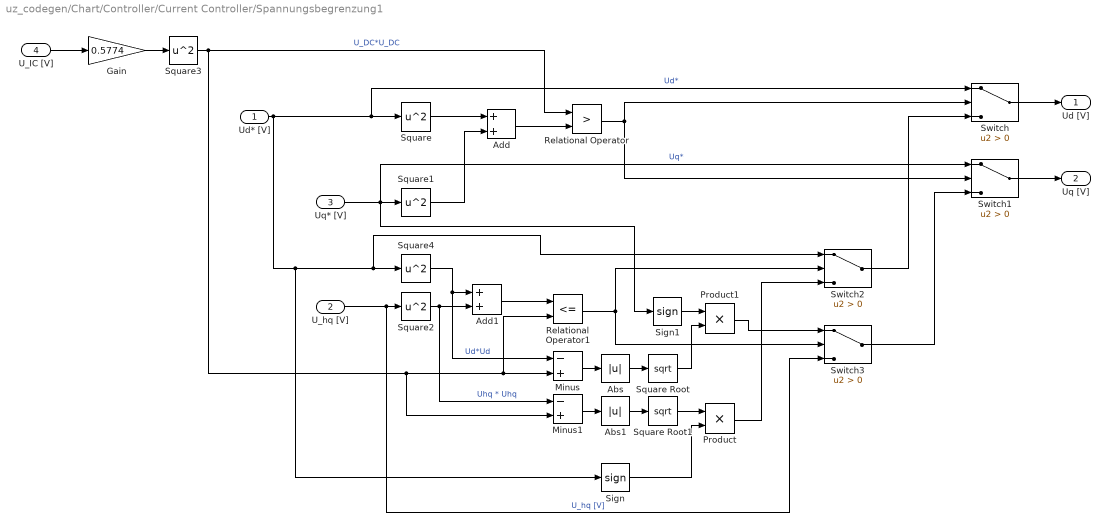
== system uz_codegen/Chart/Controller/Current Controller/Spannungsbegrenzung1 ==
  Ud* [V] : Inport
  U_hq [V] : Inport  Port=2
  Uq* [V] : Inport  Port=3
  U_IC [V] : Inport  Port=4
  Abs : Abs
  Abs1 : Abs
  Add : Sum
  Add1 : Sum
  Gain : Gain  Gain=0.5774
  Minus : Sum  Inputs=-+
  Minus1 : Sum  Inputs=-+
  Product : Product
  Product1 : Product
  Relational Operator : RelationalOperator  Operator=>  OutDataTypeStr=boolean  RndMeth=Simplest
  Relational Operator1 : RelationalOperator  Operator=<=  OutDataTypeStr=boolean  RndMeth=Simplest
  Sign : Signum
  Sign1 : Signum
  Square{,1..4} (5 alike) : Math  Operator=square  SaturateOnIntegerOverflow=on
  Square Root : Sqrt  SaturateOnIntegerOverflow=on
  Square Root1 : Sqrt  SaturateOnIntegerOverflow=on
  Switch{,1..3} (4 alike) : Switch  Criteria=u2 > Threshold
  Ud [V] : Outport
  Uq [V] : Outport  Port=2
  wires:
  Ud* [V]/1 -> Sign/1, Switch2/1, Square4/1, Switch/1, Square/1  "Ud*"
  Uq* [V]/1 -> Switch1/1, Sign1/1, Square1/1  "Uq*"
  U_hq [V]/1 -> Switch3/3, Square2/1  "U_hq [V]"
  U_IC [V]/1 -> Gain/1
  Square1/1 -> Add/2
  Square/1 -> Add/1
  Square3/1 -> Minus1/2, Minus/2, Relational Operator1/2, Relational Operator/1  "U_DC*U_DC"
  Add/1 -> Relational Operator/2
  Switch/1 -> Ud [V]/1
  Relational Operator/1 -> Switch1/2, Switch/2
  Switch1/1 -> Uq [V]/1
  Square2/1 -> Minus1/1, Add1/2  "Uhq * Uhq"
  Square4/1 -> Minus/1, Add1/1  "Ud*Ud"
  Add1/1 -> Relational Operator1/1
  Relational Operator1/1 -> Switch2/2, Switch3/2
  Switch2/1 -> Switch/3
  Switch3/1 -> Switch1/3
  Minus/1 -> Abs/1
  Square Root/1 -> Product1/2
  Minus1/1 -> Abs1/1
  Square Root1/1 -> Product/1
  Abs1/1 -> Square Root1/1
  Abs/1 -> Square Root/1
  Gain/1 -> Square3/1
  Sign/1 -> Product/2
  Product/1 -> Switch2/3
  Sign1/1 -> Product1/1
  Product1/1 -> Switch3/1

== system uz_codegen/Chart/Controller/speed controller/MMPA_Controller ==
  flg_speedControl : Inport
  n_soll : Inport  Port=2
  n_ist : Inport  Port=3
  id_ref : Inport  Port=4
  iq_ref : Inport  Port=5
  Discrete Transfer Fcn : DiscreteTransferFcn  Numerator=num_Gd_trq  Denominator=denum_Gd_trq
  PID Controller : pid_lib/PID Controller  Controller=PI  Form=Ideal  TimeDomain=Discrete-time  UseExternalTs=off  SampleTime=-1  IntegratorMethod=Forward Euler  FilterMethod=Forward Euler  ControllerParametersSource=internal  P=Kp_TorqueController  I=Ki_TorqueController  D=0  UseFilter=on  N=100  TunerSelectOption=Transfer Function Based (PID Tuner App)  InitialConditionSource=internal  InitialConditionForIntegrator=0  InitialConditionForFilter=0  DifferentiatorICPrevScaledInput=0  ExternalReset=none  TrackingMode=off  Kt=1  LimitOutput=on  SatLimitsSource=internal  UpperSaturationLimit=8  LowerSaturationLimit=-8  LinearizeAsGain=on  AntiWindupMode=clamping  Kb=1  POutMin=[]  POutMax=[]  IOutMin=[]  IOutMax=[]  DOutMin=[]  DOutMax=[]  NOutMin=[]  NOutMax=[]  SumOutMin=[]  SumOutMax=[]  SaturationOutMin=[]  SaturationOutMax=[]  PParamMin=[]  PParamMax=[]  IParamMin=[]  IParamMax=[]  DParamMin=[]  DParamMax=[]  NParamMin=[]  NParamMax=[]  KbParamMin=[]  KbParamMax=[]  KtParamMin=[]  KtParamMax=[]  KbOutMin=[]  KbOutMax=[]  KtOutMin=[]  KtOutMax=[]  IntegratorOutMin=[]  IntegratorOutMax=[]  FilterOutMin=[]  FilterOutMax=[]  SumI1OutMin=[]  SumI1OutMax=[]  SumI2OutMin=[]  SumI2OutMax=[]  SumI3OutMin=[]  SumI3OutMax=[]  SumI4OutMin=[]  SumI4OutMax=[]  SumDOutMin=[]  SumDOutMax=[]  DifferentiatorOutMin=[]  DifferentiatorOutMax=[]  FilterDiffOutCoefMin=[]  FilterDiffOutCoefMax=[]  ReciprocalOutMin=[]  ReciprocalOutMax=[]  SumDenOutMin=[]  SumDenOutMax=[]  SumNumOutMin=[]  SumNumOutMax=[]  DivideOutMin=[]  DivideOutMax=[]  UdiffTsProdOutMin=[]  UdiffTsProdOutMax=[]  NTsProdOutMin=[]  NTsProdOutMax=[]  UintegralTsProdOutMin=[]  UintegralTsProdOutMax=[]  UngainTsProdOutMin=[]  UngainTsProdOutMax=[]  IntegratorContinuousStateAttributes=''  IntegratorStateMustResolveToSignalObject=off  IntegratorRTWStateStorageClass=Auto  FilterContinuousStateAttributes=''  FilterStateMustResolveToSignalObject=off  FilterRTWStateStorageClass=Auto  ParallelPVariant=Passthrough  IdealPVariant=InternalParameters  IVariant=InternalParameters  DVariant=Disabled  IntegratorVariant=Discrete  SatVariant=Enabled  AWVariant=DiscClampingIdeal  PCopyVariant=InternalParamsIdeal  TRVariant=Disabled  FdbkBlocksVariant=Forward  IdealPFdbkVariant=Disabled  SatFdbkVariant=Disabled  DerivativeFilterVariant=Disabled  NVariant=Disabled  NCopyVariant=Disabled_SignalSpec  FilterICVariant=Disabled  IntegratorICVariant=InternalICs  ExternalResetVariant=Disabled  TRSumVariant=Passthrough  SumFdbkVariant=Disabled  SumVariant=Sum_PI  TsampFilterVariant=InternalTs  TsampNgainVariant=Passthrough  TsampIntegralVariant=Passthrough  ExternalSaturationOutDataTypeStr=Inherit: Same as second input
  Scope : Scope  NumInputPorts=2
  Scope1 : Scope
  Subsystem : Subsystem
  Sum : Sum  Inputs=|+-
  Switch : Switch  Criteria=u2 > Threshold
  Switch1 : Switch  Criteria=u2 > Threshold
  id_soll : Outport
  Iq_soll : Outport  Port=2
  wires:
  Subsystem/1(Iq) -> Scope/1, Switch1/1
  PID Controller/1 -> Scope1/1, Subsystem/1(M_soll)  "M_soll"
  n_soll/1 -> Discrete Transfer Fcn/1
  flg_speedControl/1 -> Switch/2, Switch1/2
  n_ist/1 -> Sum/2, Subsystem/2(n_ist)
  iq_ref/1 -> Switch1/3
  id_ref/1 -> Switch/3
  Sum/1 -> PID Controller/1
  Subsystem/2(Id) -> Scope/2, Switch/1
  Discrete Transfer Fcn/1 -> Sum/1
  Switch1/1 -> Iq_soll/1
  Switch/1 -> id_soll/1

== system uz_codegen/Chart/Controller/speed controller/Subsystem ==
  flg_fieldWeakening : Inport
  id_ref : Inport  Port=2
  n_soll : Inport  Port=3
  flg_speedControl : Inport  Port=4
  n_ist : Inport  Port=5
  iq_ref : Inport  Port=6
  Discrete Filter : DiscreteTransferFcn  Numerator=num_Gd_speed  Denominator=denum_Gd_speed  OutMin=[-U_DC]  OutMax=[U_DC]
  Feldschwaechung : Subsystem
  PID Controller : pid_lib/PID Controller  Controller=PI  Form=Ideal  TimeDomain=Discrete-time  UseExternalTs=off  SampleTime=-1  IntegratorMethod=Forward Euler  FilterMethod=Forward Euler  ControllerParametersSource=internal  P=Kp_SpeedController  I=Ki_SpeedController  D=0  UseFilter=on  N=100  TunerSelectOption=Transfer Function Based (PID Tuner App)  InitialConditionSource=internal  InitialConditionForIntegrator=0  InitialConditionForFilter=0  DifferentiatorICPrevScaledInput=0  ExternalReset=none  TrackingMode=off  Kt=1  LimitOutput=on  SatLimitsSource=internal  UpperSaturationLimit=I_max  LowerSaturationLimit=-I_max  LinearizeAsGain=on  AntiWindupMode=clamping  Kb=1  POutMin=[]  POutMax=[]  IOutMin=[]  IOutMax=[]  DOutMin=[]  DOutMax=[]  NOutMin=[]  NOutMax=[]  SumOutMin=[]  SumOutMax=[]  SaturationOutMin=[]  SaturationOutMax=[]  PParamMin=[]  PParamMax=[]  IParamMin=[]  IParamMax=[]  DParamMin=[]  DParamMax=[]  NParamMin=[]  NParamMax=[]  KbParamMin=[]  KbParamMax=[]  KtParamMin=[]  KtParamMax=[]  KbOutMin=[]  KbOutMax=[]  KtOutMin=[]  KtOutMax=[]  IntegratorOutMin=[]  IntegratorOutMax=[]  FilterOutMin=[]  FilterOutMax=[]  SumI1OutMin=[]  SumI1OutMax=[]  SumI2OutMin=[]  SumI2OutMax=[]  SumI3OutMin=[]  SumI3OutMax=[]  SumI4OutMin=[]  SumI4OutMax=[]  SumDOutMin=[]  SumDOutMax=[]  DifferentiatorOutMin=[]  DifferentiatorOutMax=[]  FilterDiffOutCoefMin=[]  FilterDiffOutCoefMax=[]  ReciprocalOutMin=[]  ReciprocalOutMax=[]  SumDenOutMin=[]  SumDenOutMax=[]  SumNumOutMin=[]  SumNumOutMax=[]  DivideOutMin=[]  DivideOutMax=[]  UdiffTsProdOutMin=[]  UdiffTsProdOutMax=[]  NTsProdOutMin=[]  NTsProdOutMax=[]  UintegralTsProdOutMin=[]  UintegralTsProdOutMax=[]  UngainTsProdOutMin=[]  UngainTsProdOutMax=[]  IntegratorContinuousStateAttributes=''  IntegratorStateMustResolveToSignalObject=off  IntegratorRTWStateStorageClass=Auto  FilterContinuousStateAttributes=''  FilterStateMustResolveToSignalObject=off  FilterRTWStateStorageClass=Auto  ParallelPVariant=Passthrough  IdealPVariant=InternalParameters  IVariant=InternalParameters  DVariant=Disabled  IntegratorVariant=Discrete  SatVariant=Enabled  AWVariant=DiscClampingIdeal  PCopyVariant=InternalParamsIdeal  TRVariant=Disabled  FdbkBlocksVariant=Forward  IdealPFdbkVariant=Disabled  SatFdbkVariant=Disabled  DerivativeFilterVariant=Disabled  NVariant=Disabled  NCopyVariant=Disabled_SignalSpec  FilterICVariant=Disabled  IntegratorICVariant=InternalICs  ExternalResetVariant=Disabled  TRSumVariant=Passthrough  SumFdbkVariant=Disabled  SumVariant=Sum_PI  TsampFilterVariant=InternalTs  TsampNgainVariant=Passthrough  TsampIntegralVariant=Passthrough  ExternalSaturationOutDataTypeStr=Inherit: Same as second input
  Sum : Sum  Inputs=|+-
  Switch : Switch  Criteria=u2 > Threshold
  Switch1 : Switch  Criteria=u2 > Threshold
  id_soll : Outport
  iq_soll : Outport  Port=2
  wires:
  iq_ref/1 -> Switch1/3
  n_ist/1 -> Feldschwaechung/1(n_mech_soll [rpm]), Sum/2
  id_ref/1 -> Switch/3
  Feldschwaechung/1(Id_soll [A]) -> Switch/1
  flg_fieldWeakening/1 -> Switch/2
  PID Controller/1 -> Switch1/1, Feldschwaechung/2(Iq_soll [A])
  Sum/1 -> PID Controller/1
  flg_speedControl/1 -> Switch1/2
  Discrete Filter/1 -> Sum/1
  Switch/1 -> id_soll/1
  Switch1/1 -> iq_soll/1
  n_soll/1 -> Discrete Filter/1

== system uz_codegen/Chart/CurrentController/Current Controller/EntkopplungUndVorsteuerung ==
  Id_soll : Inport
  w_el [rad/s] : Inport  Port=2
  Iq_soll : Inport  Port=3
  Add : Sum
  Constant : Constant  Value=psi_pm
  Gain1 : Gain  Gain=-Lq
  Gain2 : Gain  Gain=Ld
  Product : Product
  Product1 : Product
  Product2 : Product
  Ud_entk : Outport
  Uq_ind : Outport  Port=2
  Uq_entk : Outport  Port=3
  wires:
  w_el [rad/s]/1 -> Product2/2, Product1/2, Product/1  "w_el [rad/s]"
  Iq_soll/1 -> Gain1/1
  Gain1/1 -> Product/2
  Product/1 -> Ud_entk/1  "-w_el * Iq * Lq"
  Id_soll/1 -> Gain2/1
  Gain2/1 -> Add/2
  Constant/1 -> Product2/1, Add/1
  Add/1 -> Product1/1
  Product1/1 -> Uq_entk/1  "w_el * (psi_pm + Ld * Id)"
  Product2/1 -> Uq_ind/1

== system uz_codegen/Chart/CurrentController/Current Controller/Id-Controller ==
  Id_soll : Inport
  Id_ist : Inport  Port=2
  PID Controller : pid_lib/PID Controller  Controller=PI  Form=Ideal  TimeDomain=Discrete-time  UseExternalTs=off  SampleTime=-1  IntegratorMethod=Forward Euler  FilterMethod=Forward Euler  ControllerParametersSource=internal  P=Kp_IdController  I=Ki_IdController  D=0  UseFilter=on  N=100  TunerSelectOption=Transfer Function Based (PID Tuner App)  InitialConditionSource=internal  InitialConditionForIntegrator=0  InitialConditionForFilter=0  DifferentiatorICPrevScaledInput=0  ExternalReset=none  TrackingMode=off  Kt=1  LimitOutput=on  SatLimitsSource=internal  UpperSaturationLimit=U_maxDQ  LowerSaturationLimit=-U_maxDQ  LinearizeAsGain=on  AntiWindupMode=clamping  Kb=1  POutMin=[]  POutMax=[]  IOutMin=[]  IOutMax=[]  DOutMin=[]  DOutMax=[]  NOutMin=[]  NOutMax=[]  SumOutMin=[]  SumOutMax=[]  SaturationOutMin=[]  SaturationOutMax=[]  PParamMin=[]  PParamMax=[]  IParamMin=[]  IParamMax=[]  DParamMin=[]  DParamMax=[]  NParamMin=[]  NParamMax=[]  KbParamMin=[]  KbParamMax=[]  KtParamMin=[]  KtParamMax=[]  KbOutMin=[]  KbOutMax=[]  KtOutMin=[]  KtOutMax=[]  IntegratorOutMin=[]  IntegratorOutMax=[]  FilterOutMin=[]  FilterOutMax=[]  SumI1OutMin=[]  SumI1OutMax=[]  SumI2OutMin=[]  SumI2OutMax=[]  SumI3OutMin=[]  SumI3OutMax=[]  SumI4OutMin=[]  SumI4OutMax=[]  SumDOutMin=[]  SumDOutMax=[]  DifferentiatorOutMin=[]  DifferentiatorOutMax=[]  FilterDiffOutCoefMin=[]  FilterDiffOutCoefMax=[]  ReciprocalOutMin=[]  ReciprocalOutMax=[]  SumDenOutMin=[]  SumDenOutMax=[]  SumNumOutMin=[]  SumNumOutMax=[]  DivideOutMin=[]  DivideOutMax=[]  UdiffTsProdOutMin=[]  UdiffTsProdOutMax=[]  NTsProdOutMin=[]  NTsProdOutMax=[]  UintegralTsProdOutMin=[]  UintegralTsProdOutMax=[]  UngainTsProdOutMin=[]  UngainTsProdOutMax=[]  IntegratorContinuousStateAttributes=''  IntegratorStateMustResolveToSignalObject=off  IntegratorRTWStateStorageClass=Auto  FilterContinuousStateAttributes=''  FilterStateMustResolveToSignalObject=off  FilterRTWStateStorageClass=Auto  ParallelPVariant=Passthrough  IdealPVariant=InternalParameters  IVariant=InternalParameters  DVariant=Disabled  IntegratorVariant=Discrete  SatVariant=Enabled  AWVariant=DiscClampingIdeal  PCopyVariant=InternalParamsIdeal  TRVariant=Disabled  FdbkBlocksVariant=Forward  IdealPFdbkVariant=Disabled  SatFdbkVariant=Disabled  DerivativeFilterVariant=Disabled  NVariant=Disabled  NCopyVariant=Disabled_SignalSpec  FilterICVariant=Disabled  IntegratorICVariant=InternalICs  ExternalResetVariant=Disabled  TRSumVariant=Passthrough  SumFdbkVariant=Disabled  SumVariant=Sum_PI  TsampFilterVariant=InternalTs  TsampNgainVariant=Passthrough  TsampIntegralVariant=Passthrough  ExternalSaturationOutDataTypeStr=Inherit: Same as second input
  Scope : Scope  NumInputPorts=2
  Subtract : Sum  Inputs=|+-
  Ud_ref : Outport
  wires:
  Subtract/1 -> PID Controller/1  "error"
  Id_soll/1 -> Scope/1, Subtract/1  "id_soll"
  Id_ist/1 -> Scope/2, Subtract/2  "id_ist"
  PID Controller/1 -> Ud_ref/1

== system uz_codegen/Chart/CurrentController/Current Controller/Iq-Controller ==
  Iq_ist : Inport
  Iq_soll : Inport  Port=2
  PID Controller : pid_lib/PID Controller  Controller=PI  Form=Ideal  TimeDomain=Discrete-time  UseExternalTs=off  SampleTime=-1  IntegratorMethod=Forward Euler  FilterMethod=Forward Euler  ControllerParametersSource=internal  P=Kp_IqController  I=Ki_IqController  D=0  UseFilter=on  N=100  TunerSelectOption=Transfer Function Based (PID Tuner App)  InitialConditionSource=internal  InitialConditionForIntegrator=0  InitialConditionForFilter=0  DifferentiatorICPrevScaledInput=0  ExternalReset=none  TrackingMode=off  Kt=1  LimitOutput=on  SatLimitsSource=internal  UpperSaturationLimit=U_maxDQ  LowerSaturationLimit=-U_maxDQ  LinearizeAsGain=on  AntiWindupMode=clamping  Kb=1  POutMin=[]  POutMax=[]  IOutMin=[]  IOutMax=[]  DOutMin=[]  DOutMax=[]  NOutMin=[]  NOutMax=[]  SumOutMin=[]  SumOutMax=[]  SaturationOutMin=[]  SaturationOutMax=[]  PParamMin=[]  PParamMax=[]  IParamMin=[]  IParamMax=[]  DParamMin=[]  DParamMax=[]  NParamMin=[]  NParamMax=[]  KbParamMin=[]  KbParamMax=[]  KtParamMin=[]  KtParamMax=[]  KbOutMin=[]  KbOutMax=[]  KtOutMin=[]  KtOutMax=[]  IntegratorOutMin=[]  IntegratorOutMax=[]  FilterOutMin=[]  FilterOutMax=[]  SumI1OutMin=[]  SumI1OutMax=[]  SumI2OutMin=[]  SumI2OutMax=[]  SumI3OutMin=[]  SumI3OutMax=[]  SumI4OutMin=[]  SumI4OutMax=[]  SumDOutMin=[]  SumDOutMax=[]  DifferentiatorOutMin=[]  DifferentiatorOutMax=[]  FilterDiffOutCoefMin=[]  FilterDiffOutCoefMax=[]  ReciprocalOutMin=[]  ReciprocalOutMax=[]  SumDenOutMin=[]  SumDenOutMax=[]  SumNumOutMin=[]  SumNumOutMax=[]  DivideOutMin=[]  DivideOutMax=[]  UdiffTsProdOutMin=[]  UdiffTsProdOutMax=[]  NTsProdOutMin=[]  NTsProdOutMax=[]  UintegralTsProdOutMin=[]  UintegralTsProdOutMax=[]  UngainTsProdOutMin=[]  UngainTsProdOutMax=[]  IntegratorContinuousStateAttributes=''  IntegratorStateMustResolveToSignalObject=off  IntegratorRTWStateStorageClass=Auto  FilterContinuousStateAttributes=''  FilterStateMustResolveToSignalObject=off  FilterRTWStateStorageClass=Auto  ParallelPVariant=Passthrough  IdealPVariant=InternalParameters  IVariant=InternalParameters  DVariant=Disabled  IntegratorVariant=Discrete  SatVariant=Enabled  AWVariant=DiscClampingIdeal  PCopyVariant=InternalParamsIdeal  TRVariant=Disabled  FdbkBlocksVariant=Forward  IdealPFdbkVariant=Disabled  SatFdbkVariant=Disabled  DerivativeFilterVariant=Disabled  NVariant=Disabled  NCopyVariant=Disabled_SignalSpec  FilterICVariant=Disabled  IntegratorICVariant=InternalICs  ExternalResetVariant=Disabled  TRSumVariant=Passthrough  SumFdbkVariant=Disabled  SumVariant=Sum_PI  TsampFilterVariant=InternalTs  TsampNgainVariant=Passthrough  TsampIntegralVariant=Passthrough  ExternalSaturationOutDataTypeStr=Inherit: Same as second input
  Scope : Scope  NumInputPorts=2
  Subtract : Sum  Inputs=|+-
  Uq_ref : Outport
  wires:
  Subtract/1 -> PID Controller/1  "error"
  Iq_soll/1 -> Scope/1, Subtract/1  "iq_soll"
  Iq_ist/1 -> Scope/2, Subtract/2  "iq_ist"
  PID Controller/1 -> Uq_ref/1

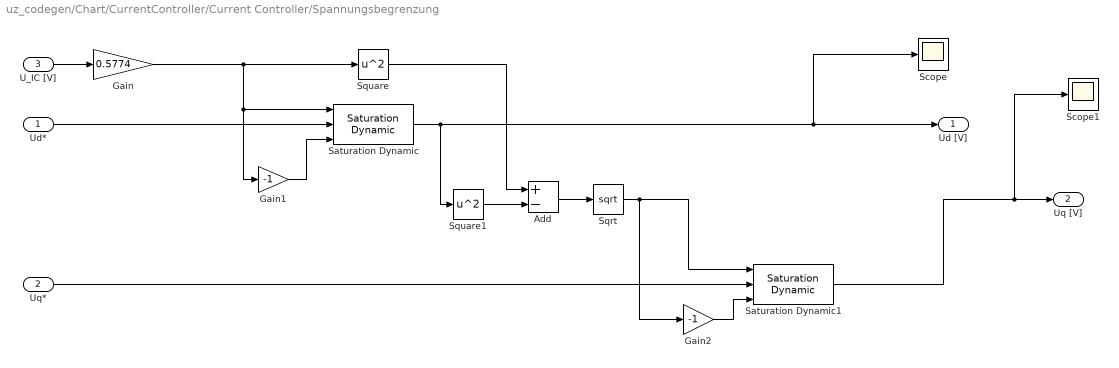
== system uz_codegen/Chart/CurrentController/Current Controller/Spannungsbegrenzung ==
  Ud* : Inport
  Uq* : Inport  Port=2
  U_IC [V] : Inport  Port=3
  Add : Sum  Inputs=+-
  Gain : Gain  Gain=0.5774
  Gain1 : Gain  Gain=-1
  Gain2 : Gain  Gain=-1
  Saturation Dynamic : simulink/Discontinuities/Saturation Dynamic  OutMin=[]  OutMax=[]  OutDataTypeStr=Inherit: Same as second input  OutDataType=fixdt(1, 16)  OutScaling=2^-10  DoSatur=off
  Saturation Dynamic1 : simulink/Discontinuities/Saturation Dynamic  OutMin=[]  OutMax=[]  OutDataTypeStr=Inherit: Same as second input  OutDataType=fixdt(1, 16)  OutScaling=2^-10  DoSatur=off
  Scope : Scope
  Scope1 : Scope
  Sqrt : Sqrt  SaturateOnIntegerOverflow=on
  Square : Math  Operator=square  SaturateOnIntegerOverflow=on
  Square1 : Math  Operator=square  SaturateOnIntegerOverflow=on
  Ud [V] : Outport
  Uq [V] : Outport  Port=2
  wires:
  Gain2/1 -> Saturation Dynamic1/3
  Add/1 -> Sqrt/1
  Square/1 -> Add/1
  Sqrt/1 -> Gain2/1, Saturation Dynamic1/1
  Saturation Dynamic/1 -> Scope/1, Ud [V]/1, Square1/1
  Saturation Dynamic1/1 -> Scope1/1, Uq [V]/1
  Gain1/1 -> Saturation Dynamic/3
  Uq*/1 -> Saturation Dynamic1/2
  U_IC [V]/1 -> Gain/1
  Gain/1 -> Square/1, Saturation Dynamic/1, Gain1/1
  Square1/1 -> Add/2
  Ud*/1 -> Saturation Dynamic/2
